simulink model "GR_Model_TT"  (R2020a)
settings: Solver=FixedStepAuto  StartTime=0.0  StopTime=100  FixedStep=0.01  RelTol=1e-3
InitFcn:
  | GR_Parameters;
values from neighbouring files (symbols this model uses):
  KP = 1    [GR_Parameters.m]
  KR = 1    [GR_Parameters.m]
  p0 = [0,0]    [GR_Parameters.m]
  R0 = [cos(psi0) -sin(psi0);        sin(psi0) cos(psi0)]    [GR_Parameters.m]
libraries: vrlib x2
settings Model: Creator=vcichella  LastModifiedBy=vcichella
settings SFSimCC: CustomCodeUndefinedFunction=UseInterfaceOnly

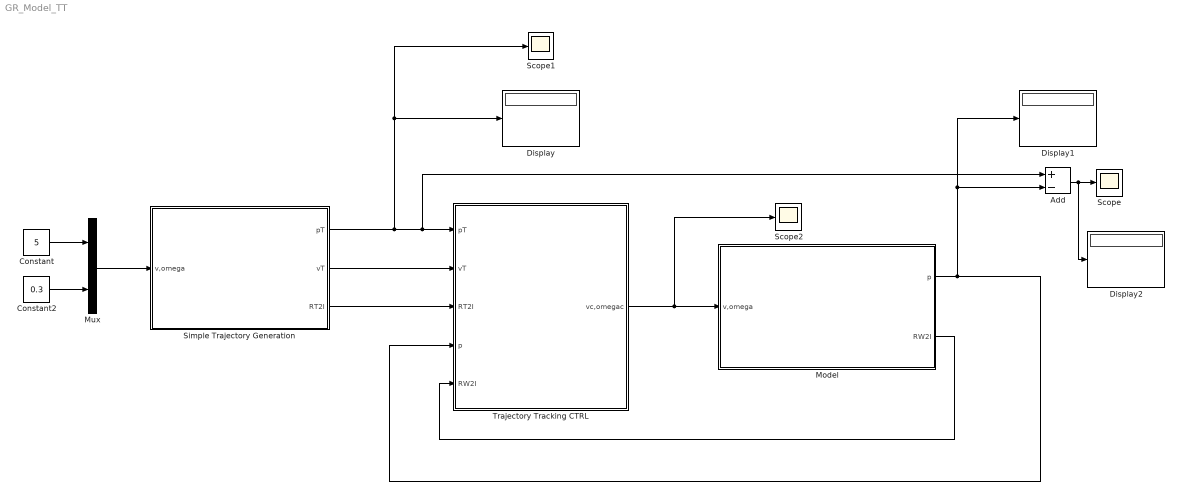
== system GR_Model_TT ==
  Add : Sum  Inputs=+-
  Constant : Constant  Value=5
  Constant2 : Constant  Value=0.3
  Display : Display
  Display1 : Display
  Display2 : Display
  Model : Subsystem
  Mux : Mux  Inputs=2
  Scope : Scope
  Scope1 : Scope
  Scope2 : Scope
  Simple Trajectory Generation : Subsystem
  "Trajectory Tracking CTRL " : Subsystem
  wires:
  Simple Trajectory Generation/3(RT2I) -> "Trajectory Tracking CTRL "/3(RT2I)
  Constant/1 -> Mux/1
  Simple Trajectory Generation/1(pT) -> Add/1, "Trajectory Tracking CTRL "/1(pT), Scope1/1, Display/1
  Mux/1 -> Simple Trajectory Generation/1(v,omega)
  Constant2/1 -> Mux/2
  Simple Trajectory Generation/2(vT) -> "Trajectory Tracking CTRL "/2(vT)
  Add/1 -> Display2/1, Scope/1
  "Trajectory Tracking CTRL "/1(vc,omegac) -> Scope2/1, Model/1(v,omega)
  Model/2(RW2I) -> "Trajectory Tracking CTRL "/5(RW2I)
  Model/1(p) -> Add/2, Display1/1, "Trajectory Tracking CTRL "/4(p)

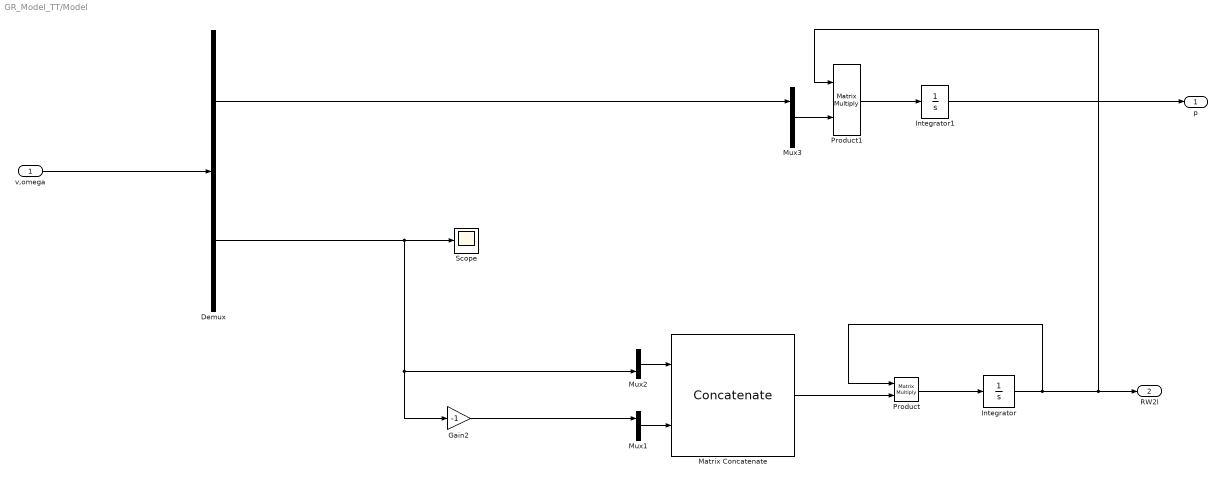
== system GR_Model_TT/Model ==
  v,omega : Inport
  Demux : Demux  Outputs=2
  Gain2 : Gain  Gain=-1
  Integrator : Integrator  InitialCondition=R0
  Integrator1 : Integrator  InitialCondition=p0
  Matrix Concatenate : Concatenate  Mode=Multidimensional array  ConcatenateDimension=2
  Mux1 : Mux  Inputs=2
  Mux2 : Mux  Inputs=2
  Mux3 : Mux  Inputs=2
  Product : Product  Multiplication=Matrix(*)
  Product1 : Product  Multiplication=Matrix(*)
  Scope : Scope
  p : Outport  VectorParamsAs1DForOutWhenUnconnected=off
  RW2I : Outport  Port=2  VectorParamsAs1DForOutWhenUnconnected=off
  wires:
  Demux/1 -> Mux3/1
  Demux/2 -> Scope/1, Mux2/2, Gain2/1
  Mux2/1 -> Matrix Concatenate/1
  Matrix Concatenate/1 -> Product/2
  v,omega/1 -> Demux/1
  Product1/1 -> Integrator1/1
  Mux3/1 -> Product1/2
  Mux1/1 -> Matrix Concatenate/2
  Integrator1/1 -> p/1
  Integrator/1 -> Product/1, RW2I/1, Product1/1
  Product/1 -> Integrator/1
  Gain2/1 -> Mux1/1

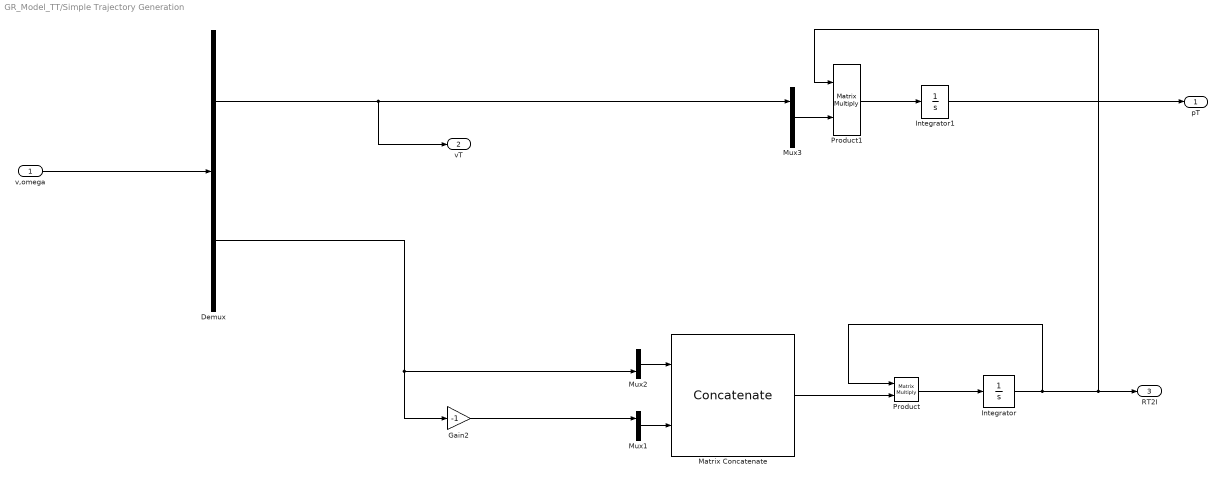
== system GR_Model_TT/Simple Trajectory Generation ==
  v,omega : Inport
  Demux : Demux  Outputs=2
  Gain2 : Gain  Gain=-1
  Integrator : Integrator  InitialCondition=R0
  Integrator1 : Integrator  InitialCondition=p0
  Matrix Concatenate : Concatenate  Mode=Multidimensional array  ConcatenateDimension=2
  Mux1 : Mux  Inputs=2
  Mux2 : Mux  Inputs=2
  Mux3 : Mux  Inputs=2
  Product : Product  Multiplication=Matrix(*)
  Product1 : Product  Multiplication=Matrix(*)
  pT : Outport  VectorParamsAs1DForOutWhenUnconnected=off
  vT : Outport  Port=2  VectorParamsAs1DForOutWhenUnconnected=off
  RT2I : Outport  Port=3  VectorParamsAs1DForOutWhenUnconnected=off
  wires:
  Mux3/1 -> Product1/2
  Integrator/1 -> Product/1, RT2I/1, Product1/1
  Product1/1 -> Integrator1/1
  Integrator1/1 -> pT/1
  Product/1 -> Integrator/1
  Mux1/1 -> Matrix Concatenate/2
  v,omega/1 -> Demux/1
  Matrix Concatenate/1 -> Product/2
  Mux2/1 -> Matrix Concatenate/1
  Demux/2 -> Mux2/2, Gain2/1
  Gain2/1 -> Mux1/1
  Demux/1 -> vT/1, Mux3/1

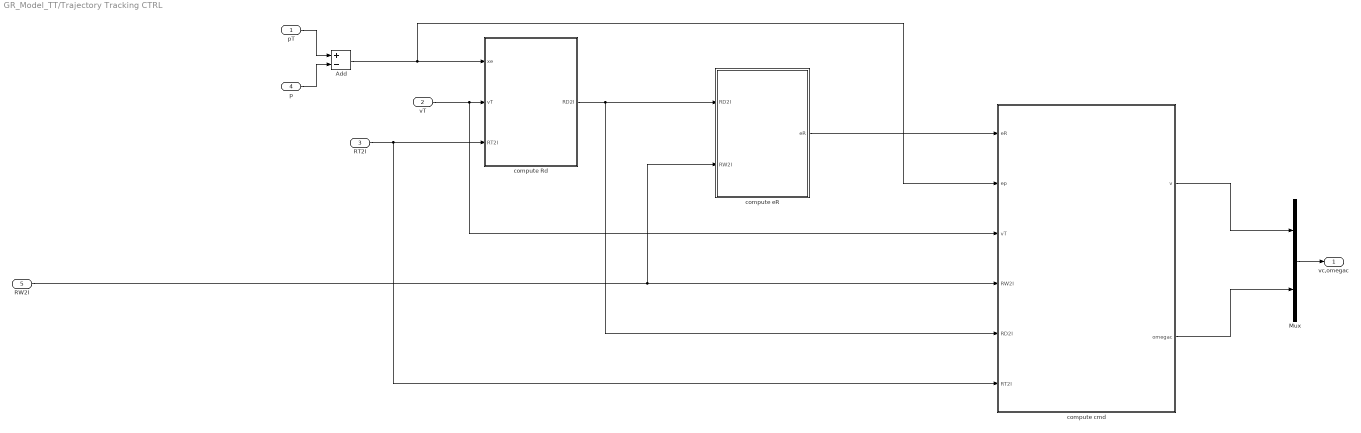
== system GR_Model_TT/Trajectory Tracking CTRL  ==
  pT : Inport
  vT : Inport  Port=2
  RT2I : Inport  Port=3
  p : Inport  Port=4
  RW2I : Inport  Port=5
  Add : Sum  Inputs=+-
  Mux : Mux  Inputs=2
  compute Rd : Subsystem
  compute cmd : Subsystem
  compute eR : Subsystem
  vc,omegac : Outport  VectorParamsAs1DForOutWhenUnconnected=off
  wires:
  pT/1 -> Add/1
  p/1 -> Add/2
  vT/1 -> compute cmd/3(vT), compute Rd/2(vT)
  RT2I/1 -> compute cmd/6(RT2I), compute Rd/3(RT2I)
  compute Rd/1(RD2I) -> compute cmd/5(RD2I), compute eR/1(RD2I)
  compute eR/1(eR) -> compute cmd/1(eR)
  Add/1 -> compute cmd/2(ep), compute Rd/1(xe)
  RW2I/1 -> compute eR/2(RW2I), compute cmd/4(RW2I)
  Mux/1 -> vc,omegac/1
  compute cmd/1("v ") -> Mux/1
  compute cmd/2(omegac) -> Mux/2

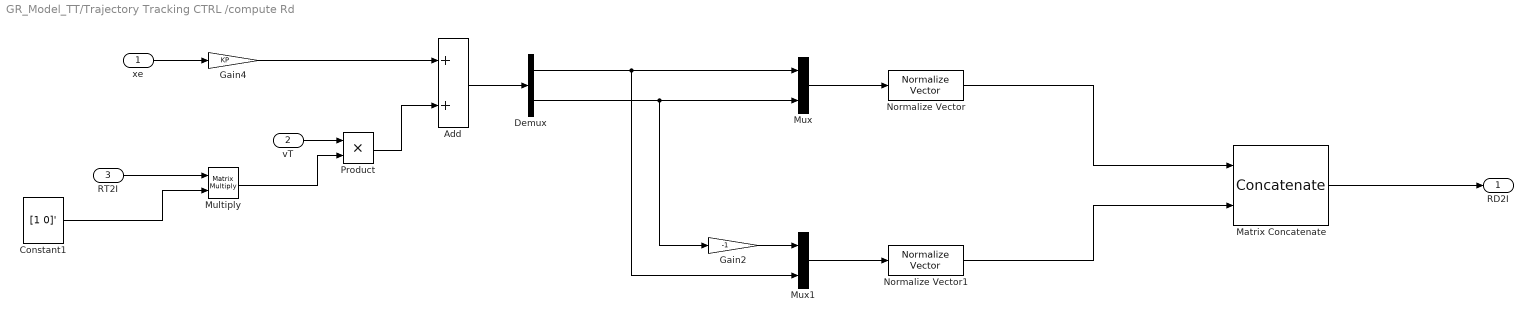
== system GR_Model_TT/Trajectory Tracking CTRL /compute Rd ==
  xe : Inport
  vT : Inport  Port=2
  RT2I : Inport  Port=3
  Add : Sum
  Constant1 : Constant  Value=[1 0]'
  Demux : Demux  Outputs=2
  Gain2 : Gain  Gain=-1
  Gain4 : Gain  Gain=KP
  Matrix Concatenate : Concatenate  Mode=Multidimensional array  ConcatenateDimension=2
  Multiply : Product  Multiplication=Matrix(*)
  Mux : Mux  Inputs=2
  Mux1 : Mux  Inputs=2
  Normalize Vector : vrlib/Utilities/Normalize Vector  maxzero=0
  Normalize Vector1 : vrlib/Utilities/Normalize Vector  maxzero=0
  Product : Product
  RD2I : Outport  VectorParamsAs1DForOutWhenUnconnected=off
  wires:
  Mux/1 -> Normalize Vector/1
  Mux1/1 -> Normalize Vector1/1
  Normalize Vector/1 -> Matrix Concatenate/1
  Normalize Vector1/1 -> Matrix Concatenate/2
  xe/1 -> Gain4/1
  Matrix Concatenate/1 -> RD2I/1
  vT/1 -> Product/1
  Product/1 -> Add/2
  Add/1 -> Demux/1
  Multiply/1 -> Product/2
  RT2I/1 -> Multiply/1
  Constant1/1 -> Multiply/2
  Gain4/1 -> Add/1
  Gain2/1 -> Mux1/1
  Demux/1 -> Mux1/2, Mux/1
  Demux/2 -> Gain2/1, Mux/2

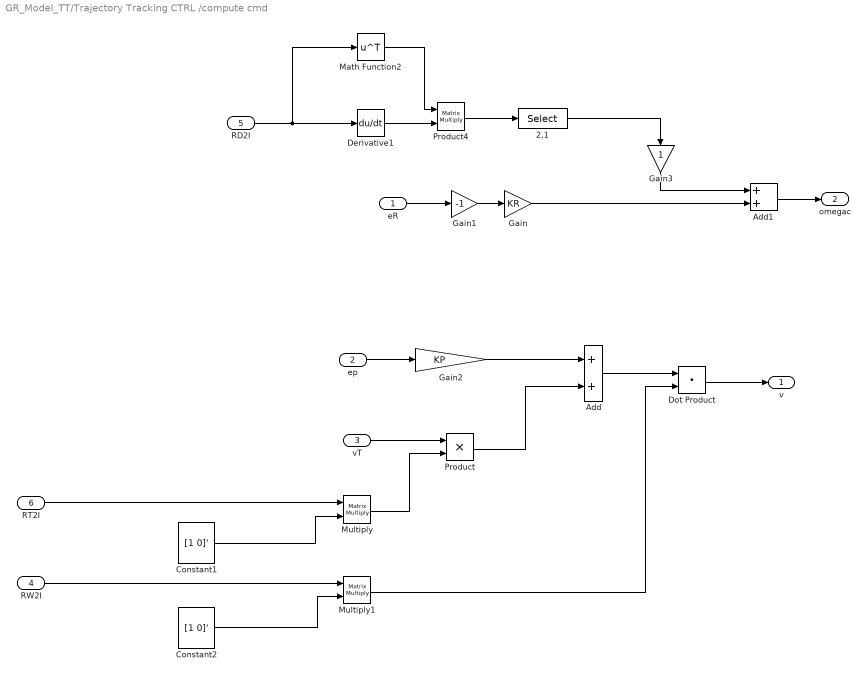
== system GR_Model_TT/Trajectory Tracking CTRL /compute cmd ==
  eR : Inport
  ep : Inport  Port=2
  vT : Inport  Port=3
  RW2I : Inport  Port=4
  RD2I : Inport  Port=5
  RT2I : Inport  Port=6
  2,1 : Selector  NumberOfDimensions=2  InputPortWidth=9  IndexOptions=Index vector (dialog),Index vector (dialog)  Indices=2,1  OutputSizes=1
  Add : Sum
  Add1 : Sum
  Constant1 : Constant  Value=[1 0]'
  Constant2 : Constant  Value=[1 0]'
  Derivative1 : Derivative
  Dot Product : DotProduct  InputSameDT=on  OutDataTypeStr=Inherit: Inherit via internal rule
  Gain : Gain  Gain=KR
  Gain1 : Gain  Gain=-1
  Gain2 : Gain  Gain=KP
  Gain3 : Gain
  Math Function2 : Math  Operator=transpose  SignedPower=on  SaturateOnIntegerOverflow=on
  Multiply : Product  Multiplication=Matrix(*)
  Multiply1 : Product  Multiplication=Matrix(*)
  Product : Product
  Product4 : Product  Multiplication=Matrix(*)  RndMeth=Zero
  "v " : Outport  VectorParamsAs1DForOutWhenUnconnected=off
  omegac : Outport  Port=2  VectorParamsAs1DForOutWhenUnconnected=off
  wires:
  eR/1 -> Gain1/1
  Gain1/1 -> Gain/1
  ep/1 -> Gain2/1
  vT/1 -> Product/1
  Multiply/1 -> Product/2
  Add/1 -> Dot Product/1
  Dot Product/1 -> "v "/1
  Multiply1/1 -> Dot Product/2
  Gain/1 -> Add1/2
  RT2I/1 -> Multiply/1
  Constant1/1 -> Multiply/2
  RW2I/1 -> Multiply1/1
  Constant2/1 -> Multiply1/2
  Gain3/1 -> Add1/1
  Math Function2/1 -> Product4/1
  2,1/1 -> Gain3/1
  Product4/1 -> 2,1/1
  Derivative1/1 -> Product4/2
  Product/1 -> Add/2
  Gain2/1 -> Add/1
  Add1/1 -> omegac/1
  RD2I/1 -> Math Function2/1, Derivative1/1

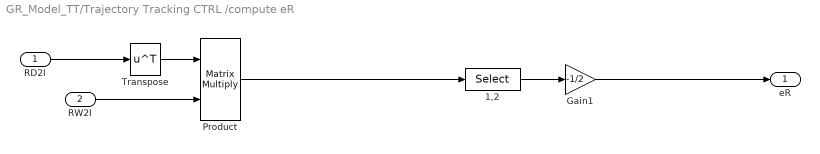
== system GR_Model_TT/Trajectory Tracking CTRL /compute eR ==
  RD2I : Inport
  RW2I : Inport  Port=2
  1,2 : Selector  NumberOfDimensions=2  InputPortWidth=9  IndexOptions=Index vector (dialog),Index vector (dialog)  Indices=1,2  OutputSizes=1
  Gain1 : Gain  Gain=-1/2
  Product : Product  Multiplication=Matrix(*)
  Transpose : Math  Operator=transpose  SignedPower=on  SaturateOnIntegerOverflow=on
  eR : Outport  VectorParamsAs1DForOutWhenUnconnected=off
  wires:
  RD2I/1 -> Transpose/1
  RW2I/1 -> Product/2
  Transpose/1 -> Product/1
  1,2/1 -> Gain1/1
  Product/1 -> 1,2/1
  Gain1/1 -> eR/1
